simulink model "Crazyflie_servo_system"  (R2020b)
settings: Solver=VariableStepAuto  StartTime=0.0  StopTime=10  RelTol=1e-3
values from neighbouring files (symbols this model uses):
  m = 0.028    [Crazyflie_get_LQ_Gain.m]
  stateA = [0  0  0  1  0  0  0  0  0  0  0  0 ... (first row only)    [Crazyflie_get_LQ_Gain.m]
  stateB = [0   0      0     0 ... (first row only)    [Crazyflie_get_LQ_Gain.m]
  stateC = eye(12)    [Crazyflie_get_LQ_Gain.m]
  stateD = zeros(12, 4)    [Crazyflie_get_LQ_Gain.m]
libraries: pid_lib x1
settings Model: Creator=kt012  LastModifiedBy=kt012
settings DebuggingCC: ArithmeticOperatorsInVariantConditions=warning
settings SFSimCC: CustomCodeUndefinedFunction=UseInterfaceOnly

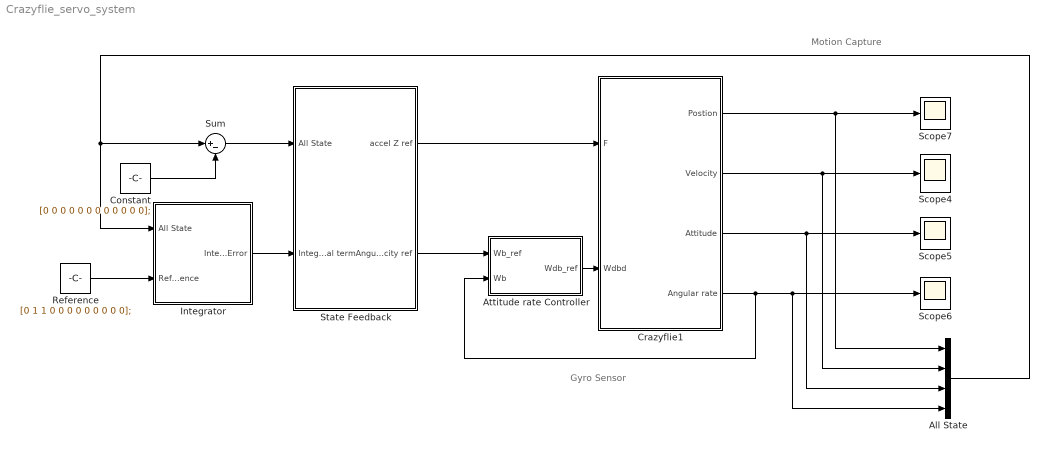
== system Crazyflie_servo_system ==
  note: Motion Capture
  note: Gyro Sensor
  All State : Mux
  Attitude rate Controller : Subsystem
  Constant : Constant  Value=[0 0 0 0 0 0 0 0 0 0 0 0];
  Crazyflie1 : Subsystem
  Integrator : Subsystem
  Reference : Constant  Value=[0 1 1 0 0 0 0 0 0 0 0 0];
  Scope{4..7} (4 alike) : Scope
  State Feedback : Subsystem
  Sum : Sum  Inputs=|+-
  wires:
  Crazyflie1/3(Attitude) -> All State/3, Scope5/1
  Crazyflie1/2(Velocity) -> All State/2, Scope4/1
  Attitude rate Controller/1(Wdb_ref) -> Crazyflie1/2(Wdbd)
  Crazyflie1/4(Angular rate) -> Attitude rate Controller/2(Wb), Scope6/1, All State/4
  State Feedback/2(Angular velocity ref) -> Attitude rate Controller/1(Wb_ref)
  Crazyflie1/1(Postion) -> All State/1, Scope7/1
  Reference/1 -> Integrator/2(Reference)
  Integrator/1(Integral Error) -> State Feedback/2(Integral term)
  State Feedback/1(accel Z ref) -> Crazyflie1/1(F)
  All State/1 -> Sum/1, Integrator/1(All State)
  Sum/1 -> State Feedback/1(All State)
  Constant/1 -> Sum/2

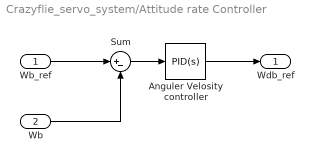
== system Crazyflie_servo_system/Attitude rate Controller ==
  Wb_ref : Inport
  Wb : Inport  Port=2
  Anguler Velosity controller : pid_lib/PID Controller  Controller=PID  Form=Parallel  TimeDomain=Continuous-time  UseExternalTs=off  SampleTime=-1  IntegratorMethod=Forward Euler  FilterMethod=Forward Euler  ControllerParametersSource=internal  P=250 * 180 / 3.14  I=500 * 180 / 3.14  D=3.0 * 180 / 3.14  UseFilter=on  N=100  TunerSelectOption=Transfer Function Based (PID Tuner App)  InitialConditionSource=internal  InitialConditionForIntegrator=0  InitialConditionForFilter=0  DifferentiatorICPrevScaledInput=0  ExternalReset=none  TrackingMode=off  Kt=1  LimitOutput=off  SatLimitsSource=internal  UpperSaturationLimit=inf  LowerSaturationLimit=-inf  LinearizeAsGain=on  AntiWindupMode=none  Kb=1  POutMin=[]  POutMax=[]  IOutMin=[]  IOutMax=[]  DOutMin=[]  DOutMax=[]  NOutMin=[]  NOutMax=[]  SumOutMin=[]  SumOutMax=[]  SaturationOutMin=[]  SaturationOutMax=[]  PParamMin=[]  PParamMax=[]  IParamMin=[]  IParamMax=[]  DParamMin=[]  DParamMax=[]  NParamMin=[]  NParamMax=[]  KbParamMin=[]  KbParamMax=[]  KtParamMin=[]  KtParamMax=[]  KbOutMin=[]  KbOutMax=[]  KtOutMin=[]  KtOutMax=[]  IntegratorOutMin=[]  IntegratorOutMax=[]  FilterOutMin=[]  FilterOutMax=[]  SumI1OutMin=[]  SumI1OutMax=[]  SumI2OutMin=[]  SumI2OutMax=[]  SumI3OutMin=[]  SumI3OutMax=[]  SumI4OutMin=[]  SumI4OutMax=[]  SumDOutMin=[]  SumDOutMax=[]  DifferentiatorOutMin=[]  DifferentiatorOutMax=[]  FilterDiffOutCoefMin=[]  FilterDiffOutCoefMax=[]  ReciprocalOutMin=[]  ReciprocalOutMax=[]  SumDenOutMin=[]  SumDenOutMax=[]  SumNumOutMin=[]  SumNumOutMax=[]  DivideOutMin=[]  DivideOutMax=[]  UdiffTsProdOutMin=[]  UdiffTsProdOutMax=[]  NTsProdOutMin=[]  NTsProdOutMax=[]  UintegralTsProdOutMin=[]  UintegralTsProdOutMax=[]  UngainTsProdOutMin=[]  UngainTsProdOutMax=[]  IntegratorContinuousStateAttributes=''  IntegratorStateMustResolveToSignalObject=off  IntegratorRTWStateStorageClass=Auto  FilterContinuousStateAttributes=''  FilterStateMustResolveToSignalObject=off  FilterRTWStateStorageClass=Auto  ParallelPVariant=InternalParameters  IdealPVariant=Disabled  IVariant=InternalParameters  DVariant=InternalParameters  IntegratorVariant=Continuous  SatVariant=Disabled  AWVariant=Passthrough  PCopyVariant=Disabled  TRVariant=Disabled  FdbkBlocksVariant=Forward  IdealPFdbkVariant=Disabled  SatFdbkVariant=Disabled  DerivativeFilterVariant=ContFilter  NVariant=InternalParameters  NCopyVariant=Disabled  FilterICVariant=InternalICsFilter  IntegratorICVariant=InternalICs  ExternalResetVariant=Disabled  TRSumVariant=Passthrough  SumFdbkVariant=Disabled  SumVariant=Sum_PID  TsampFilterVariant=InternalTs  TsampNgainVariant=Passthrough  TsampIntegralVariant=Passthrough  ExternalSaturationOutDataTypeStr=Inherit: Same as second input
  Sum : Sum  Inputs=|+-
  Wdb_ref : Outport
  wires:
  Sum/1 -> Anguler Velosity controller/1
  Anguler Velosity controller/1 -> Wdb_ref/1
  Wb/1 -> Sum/2
  Wb_ref/1 -> Sum/1

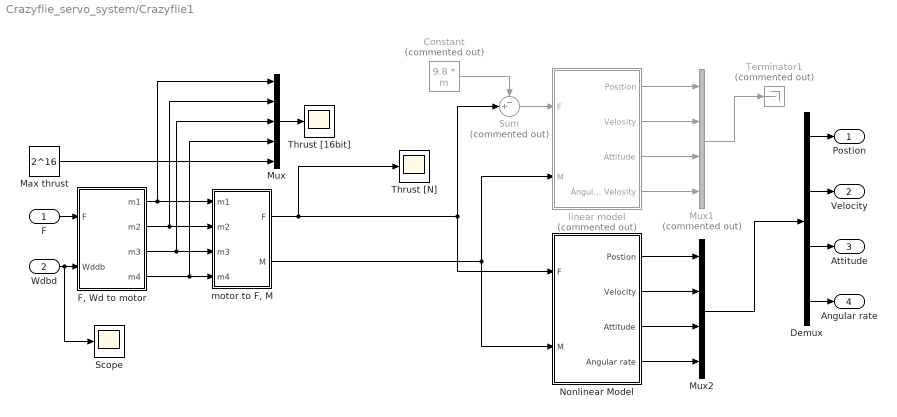
== system Crazyflie_servo_system/Crazyflie1 ==
  F : Inport
  Wdbd : Inport  Port=2
  Constant : Constant  Commented=on  Value=9.8 * m
  Demux : Demux
  "F, Wd to motor" : MATLAB Function  TreatAsAtomicUnit=on
  Max thrust : Constant  Value=2^16
  Mux : Mux  Inputs=5
  Mux1 : Mux  Commented=on
  Mux2 : Mux
  Nonlinear Model : Subsystem
  Scope : Scope
  Sum : Sum  Commented=on  Inputs=-+|
  Terminator1 : Terminator  Commented=on
  "Thrust [16bit] " : Scope
  Thrust [N] : Scope
  linear model : Subsystem  Commented=on
  "motor to F, M" : MATLAB Function  TreatAsAtomicUnit=on
  Postion : Outport
  Velocity : Outport  Port=2
  Attitude : Outport  Port=3
  Angular rate : Outport  Port=4
  wires:
  "F, Wd to motor"/1(m1) -> "motor to F, M"/1(m1), Mux/1
  Wdbd/1 -> Scope/1, "F, Wd to motor"/2(Wddb)
  "F, Wd to motor"/4(m4) -> Mux/4, "motor to F, M"/4(m4)
  "F, Wd to motor"/2(m2) -> "motor to F, M"/2(m2), Mux/2
  "F, Wd to motor"/3(m3) -> "motor to F, M"/3(m3), Mux/3
  F/1 -> "F, Wd to motor"/1(F)
  Mux/1 -> "Thrust [16bit] "/1
  Max thrust/1 -> Mux/5
  "motor to F, M"/1(F) -> Thrust [N]/1, Sum/2, Nonlinear Model/1(F)
  "motor to F, M"/2(M) -> linear model/2(M), Nonlinear Model/2(M)
  Nonlinear Model/1(Postion) -> Mux2/1
  Nonlinear Model/2(Velocity) -> Mux2/2
  Nonlinear Model/3(Attitude) -> Mux2/3
  Nonlinear Model/4(Angular rate) -> Mux2/4
  linear model/1(Position) -> Mux1/1
  linear model/2(Velosity) -> Mux1/2
  linear model/3(Attitude) -> Mux1/3
  linear model/4(Angular Velosity) -> Mux1/4
  Mux1/1 -> Terminator1/1
  Mux2/1 -> Demux/1
  Demux/1 -> Postion/1
  Demux/2 -> Velocity/1
  Demux/3 -> Attitude/1
  Demux/4 -> Angular rate/1
  Sum/1 -> linear model/1(F)
  Constant/1 -> Sum/1

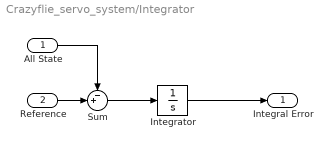
== system Crazyflie_servo_system/Integrator ==
  All State : Inport
  Reference : Inport  Port=2
  Integrator : Integrator
  Sum : Sum  Inputs=-+|
  Integral Error : Outport
  wires:
  All State/1 -> Sum/1
  Reference/1 -> Sum/2
  Sum/1 -> Integrator/1
  Integrator/1 -> Integral Error/1

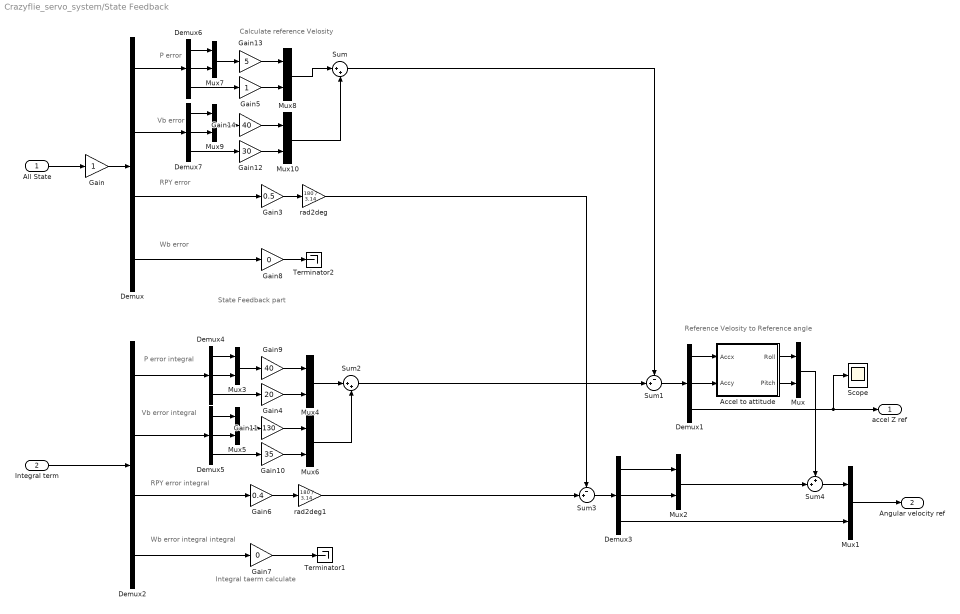
== system Crazyflie_servo_system/State Feedback ==
  note: State Feedback part
  note: P error
  note: Calculate reference Velosity
  note: Reference Velosity to Reference angle
  note: Vb error
  note: RPY error
  note: Wb error
  note: P error integral
  note: Vb error integral
  note: RPY error integral
  note: Wb error integral
      |  integral
  note: Integral taerm calculate
  All State : Inport
  Integral term : Inport  Port=2
  Accel to attitude : MATLAB Function  TreatAsAtomicUnit=on
  Demux : Demux
  Demux{1,3..7} (6 alike) : Demux  Outputs=3
  Demux2 : Demux
  Gain : Gain
  Gain10 : Gain  Gain=35
  Gain11 : Gain  Gain=130
  Gain12 : Gain  Gain=30
  Gain13 : Gain  Gain=5
  Gain14 : Gain  Gain=40
  Gain3 : Gain  Gain=0.5
  Gain4 : Gain  Gain=20
  Gain5 : Gain
  Gain6 : Gain  Gain=0.4
  Gain7 : Gain  Gain=0
  Gain8 : Gain  Gain=0
  Gain9 : Gain  Gain=40
  Mux{,1..10} (11 alike) : Mux  Inputs=2
  Scope : Scope
  Sum : Sum  Inputs=|++
  Sum1 : Sum  Inputs=-+|
  Sum2 : Sum  Inputs=|++
  Sum3 : Sum  Inputs=-+|
  Sum4 : Sum  Inputs=++|
  Terminator1 : Terminator
  Terminator2 : Terminator
  rad2deg : Gain  Gain=180 / 3.14
  rad2deg1 : Gain  Gain=180 / 3.14
  accel Z ref : Outport
  Angular velocity ref : Outport  Port=2
  wires:
  All State/1 -> Gain/1
  Gain/1 -> Demux/1
  Demux/3 -> Gain3/1
  Demux/4 -> Gain8/1
  Mux10/1 -> Sum/2
  Sum/1 -> Sum1/1
  Demux1/3 -> accel Z ref/1, Scope/1
  Gain3/1 -> rad2deg/1
  Integral term/1 -> Demux2/1
  Demux2/1 -> Demux4/1
  Demux2/2 -> Demux5/1
  Demux2/4 -> Gain7/1
  Sum1/1 -> Demux1/1
  Sum2/1 -> Sum1/2
  Demux1/1 -> Accel to attitude/1(Accx)
  Demux1/2 -> Accel to attitude/2(Accy)
  Accel to attitude/2(Pitch) -> Mux/2
  Accel to attitude/1(Roll) -> Mux/1
  Mux/1 -> Sum4/1
  Sum3/1 -> Demux3/1
  Sum4/1 -> Mux1/1
  Demux2/3 -> Gain6/1
  Demux3/1 -> Mux2/1
  Demux3/2 -> Mux2/2
  Mux2/1 -> Sum4/2
  Demux3/3 -> Mux1/2
  Gain6/1 -> rad2deg1/1
  Gain4/1 -> Mux4/2
  Mux6/1 -> Sum2/2
  Gain7/1 -> Terminator1/1
  Gain8/1 -> Terminator2/1
  Mux1/1 -> Angular velocity ref/1
  Demux4/1 -> Mux3/1
  Demux4/2 -> Mux3/2
  Demux4/3 -> Gain4/1
  Mux3/1 -> Gain9/1
  Gain9/1 -> Mux4/1
  Mux4/1 -> Sum2/1
  rad2deg/1 -> Sum3/1
  rad2deg1/1 -> Sum3/2
  Gain11/1 -> Mux6/1
  Mux5/1 -> Gain11/1
  Demux5/3 -> Gain10/1
  Demux5/2 -> Mux5/2
  Demux5/1 -> Mux5/1
  Gain10/1 -> Mux6/2
  Mux8/1 -> Sum/1
  Gain13/1 -> Mux8/1
  Mux7/1 -> Gain13/1
  Demux6/3 -> Gain5/1
  Demux6/2 -> Mux7/2
  Demux6/1 -> Mux7/1
  Gain5/1 -> Mux8/2
  Demux/1 -> Demux6/1
  Demux/2 -> Demux7/1
  Gain12/1 -> Mux10/2
  Demux7/1 -> Mux9/1
  Demux7/2 -> Mux9/2
  Demux7/3 -> Gain12/1
  Mux9/1 -> Gain14/1
  Gain14/1 -> Mux10/1

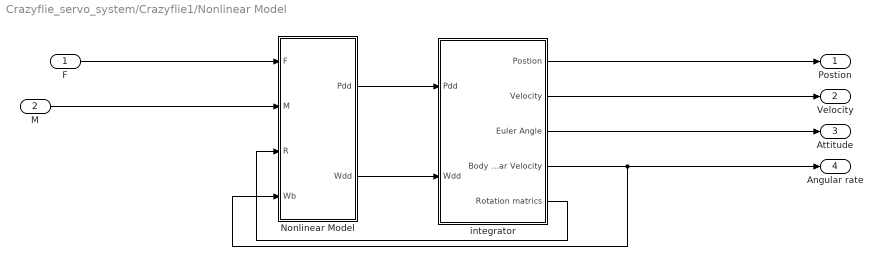
== system Crazyflie_servo_system/Crazyflie1/Nonlinear Model ==
  F : Inport
  M : Inport  Port=2
  Nonlinear Model : MATLAB Function  TreatAsAtomicUnit=on
  integrator : Subsystem
  Postion : Outport
  Velocity : Outport  Port=2
  Attitude : Outport  Port=3
  Angular rate : Outport  Port=4
  wires:
  integrator/4(Body Angular Velocity) -> Angular rate/1, Nonlinear Model/4(Wb)
  integrator/3(Euler Angle) -> Attitude/1
  Nonlinear Model/1(Pdd) -> integrator/1(Pdd)
  Nonlinear Model/2(Wdd) -> integrator/2(Wdd)
  integrator/2(Velocity) -> Velocity/1
  M/1 -> Nonlinear Model/2(M)
  integrator/1(Postion) -> Postion/1
  F/1 -> Nonlinear Model/1(F)
  integrator/5(Rotation matrics) -> Nonlinear Model/3(R)

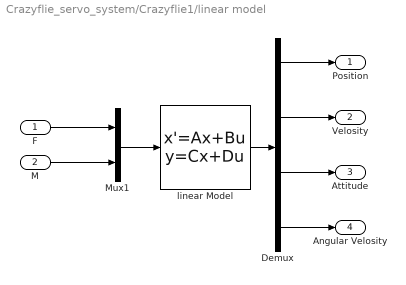
== system Crazyflie_servo_system/Crazyflie1/linear model ==
  F : Inport
  M : Inport  Port=2
  Demux : Demux
  Mux1 : Mux  Inputs=2
  linear Model : StateSpace  A=stateA  B=stateB  C=stateC  D=stateD  InitialCondition=[0 0 1 0 0 0 0 0 0 0 0 0];
  Position : Outport
  Velosity : Outport  Port=2
  Attitude : Outport  Port=3
  Angular Velosity : Outport  Port=4
  wires:
  linear Model/1 -> Demux/1
  Mux1/1 -> linear Model/1
  F/1 -> Mux1/1
  Demux/2 -> Velosity/1
  Demux/1 -> Position/1
  Demux/3 -> Attitude/1
  M/1 -> Mux1/2
  Demux/4 -> Angular Velosity/1

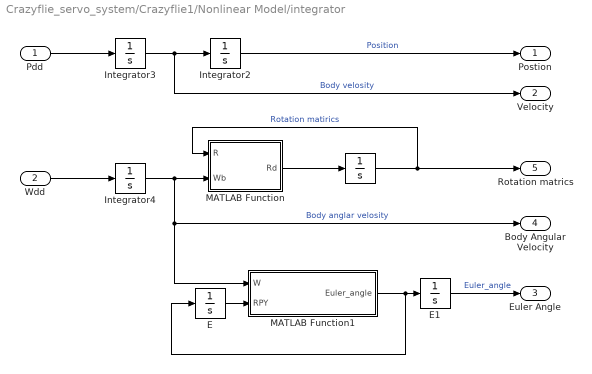
== system Crazyflie_servo_system/Crazyflie1/Nonlinear Model/integrator ==
  Pdd : Inport
  Wdd : Inport  Port=2
  " " : Integrator  InitialCondition=[1 0 0; 0 1 0; 0 0 1];  ContinuousStateAttributes="\"\""
  E : Integrator  InitialCondition=[0 0 0];
  E1 : Integrator  InitialCondition=[0 0 0];
  Integrator2 : Integrator  InitialCondition=[0 0 0];
  Integrator3 : Integrator  InitialCondition=[0 0 0.0];
  Integrator4 : Integrator  InitialCondition=[0 0 0];  ContinuousStateAttributes='Body_anglar_velocity'
  MATLAB Function : MATLAB Function  TreatAsAtomicUnit=on
  MATLAB Function1 : MATLAB Function  TreatAsAtomicUnit=on
  Postion : Outport
  Velocity : Outport  Port=2
  Euler Angle : Outport  Port=3
  Body Angular Velocity : Outport  Port=4
  Rotation matrics : Outport  Port=5
  wires:
  Integrator4/1 -> Body Angular Velocity/1, MATLAB Function1/1(W), MATLAB Function/2(Wb)  "Body anglar velosity"
  Pdd/1 -> Integrator3/1
  Integrator3/1 -> Integrator2/1, Velocity/1  "Body velosity"
  Integrator2/1 -> Postion/1  "Position"
  Wdd/1 -> Integrator4/1
  " "/1 -> MATLAB Function/1(R), Rotation matrics/1  "Rotation matirics"
  MATLAB Function/1(Rd) -> " "/1
  E/1 -> MATLAB Function1/2(RPY)
  MATLAB Function1/1(Euler_angle) -> E/1, E1/1
  E1/1 -> Euler Angle/1  "Euler_angle"

== matlab function Crazyflie_servo_system/Crazyflie1/Nonlinear Model/Nonlinear Model ==
  data: Pdd output; F input; M input; R input; Wb input; Wdd output
function [Pdd,Wdd] = fcn(F, M, R, Wb)
m = 0.035;
e3 = [0 0 1]';
g = 9.8;
% % crazyflie
I = [16.571710 0.830806 0.718277;
     0.830806 16.655602 1.800197;
     0.718277 1.800197 29.261652] * 10^(-6);      % crazyflieの慣性モーメント（kg・m^2）
% I = [1 0 0;
%      0 1 0;
%      0 0 1] * 10^(-6);
% 機体上向き加速度
Pdd = (R*F*e3 - m*g*e3)/m;

% 各加速度計算（ボディー座標系）
Wdd = pinv(I)*(M - cross(Wb, I * Wb));

== matlab function Crazyflie_servo_system/Crazyflie1/Nonlinear Model/integrator/MATLAB Function ==
  data: R input; Rd output; Wb input
function Rd = fcn(R, Wb)
wx = Wb(1);
wy = Wb(2);
wz = Wb(3);
Wb = [ 0    -wz   wy;
       wz    0   -wx;
      -wy    wx   0];
Rd = R * Wb;

== matlab function Crazyflie_servo_system/Crazyflie1/F, Wd to motor ==
  data: F input; Wddb input; m1 output; m2 output; m3 output; m4 output
 function [m1, m2, m3, m4]= fcn(F, Wddb)

% F [16bit] Wddb [16bit]
F = F * 1000 + 28000;

r = min(max(-32000, Wddb(1)), 32000)/2;
p = min(max(-32000, Wddb(2)), 32000)/2;
y = min(max(-32000, Wddb(3)), 32000);

m1 = min(max(0,F - r - p + y), 2^16);
m2 = min(max(0,F - r + p - y), 2^16);
m3 = min(max(0,F + r + p + y), 2^16);
m4 = min(max(0,F + r - p - y), 2^16);

% formation +
% r = min(max(-32000, Wddb(1)), 32000);
% p = min(max(-32000, Wddb(2)), 32000);
% y = min(max(-32000, Wddb(3)), 32000);
% m1 = min(max(0, + p + y), 2^16);
% m2 = min(max(0, - r - y), 2^16);
% m3 = min(max(0, - p + y), 2^16);
% m4 = min(max(0, + r - y), 2^16);

%         ^y
%         |
%         |
%   m3          m4
%
%                    ------>x
%
%   m2          m1

== matlab function Crazyflie_servo_system/Crazyflie1/Nonlinear Model/integrator/MATLAB Function1 ==
  data: W input; Euler_angle output; RPY input
function Euler_angle = fcn(W, RPY)
roll = RPY(1);
pitch = RPY(2);
yaw = RPY(3);
rollS = sin(roll); rollC = cos(roll);           
pitchS = sin(pitch); pitchC = cos(pitch);       


Euler_angle = pinv([1 0 -pitchS;
     0 rollC  pitchC * rollS;
     0 -rollS pitchC * rollC]) * W;

== matlab function Crazyflie_servo_system/Crazyflie1/motor to F, M ==
  data: F output; m1 input; m2 input; M output; m3 input; m4 input
function [F, M] = func(m1, m2, m3, m4)

% F [16bit] Wddb [16bit]

Armlength = 0.092/2;
m1 = 2.130295 * 10^(-11) * m1^2 + 1.032633 * 10^(-6) * m1 + 5.484560 * 10^(-4);
m2 = 2.130295 * 10^(-11) * m2^2 + 1.032633 * 10^(-6) * m2 + 5.484560 * 10^(-4);
m3 = 2.130295 * 10^(-11) * m3^2 + 1.032633 * 10^(-6) * m3 + 5.484560 * 10^(-4);
m4 = 2.130295 * 10^(-11) * m4^2 + 1.032633 * 10^(-6) * m4 + 5.484560 * 10^(-4);

% calculate thrust
F = m1 + m2 + m3 + m4;

% calculate moment formation X
M1 = Armlength / sqrt(2) * (m3 + m4 - m1 - m2);
M2 = -Armlength / sqrt(2) * (-m3 - m2 + m1 + m4);

% calculate moment formation + 
% M1 = Armlength  * (m4 - m2);
% M2 = Armlength * (m1 - m3);

M3 = m1 + m3 - m2 - m4;

M = [M1 M2 M3]';

== matlab function Crazyflie_servo_system/State Feedback/Accel to attitude ==
  data: Accx input; Roll output; Pitch output; Accy input
function [Roll, Pitch]= fcn(Accx, Accy)

Roll = -Accy * 3.14 / 180;
Pitch = -Accx * 3.14 / 180;
